simulink model "controller"  (R2021b)
settings: Solver=FixedStepAuto  StartTime=0.0  StopTime=inf  FixedStep=1/1000  RelTol=1e-3
libraries: simulink x2
settings Model: Creator=antonio  LastModifiedBy=antonio
settings OptimizationCC: DefaultUnderspecifiedDataType=single
settings ConfigComp: CovEnable=on  RecordCoverage=on  CovModelRefEnable=on

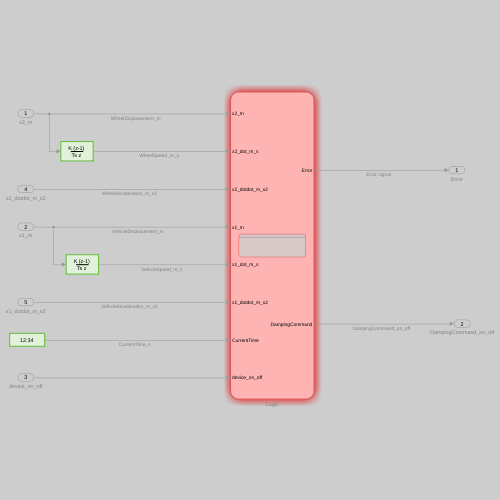
[thumbnail: Simulink's stored preview of the top-level diagram]
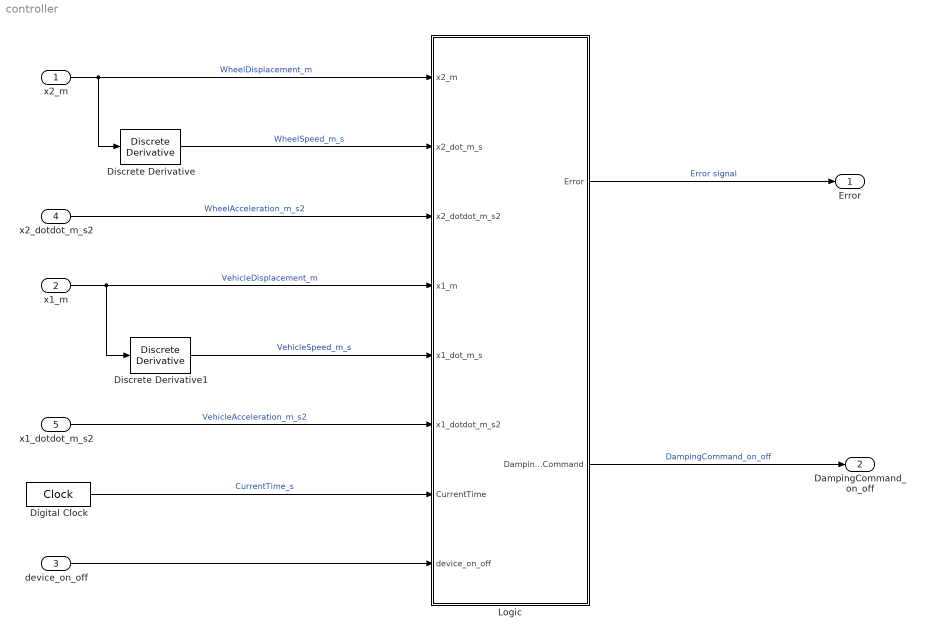
== system controller ==
  x2_m : Inport  OutDataTypeStr=double
  x1_m : Inport  Port=2
  device_on_off : Inport  Port=3
  x2_dotdot_m_s2 : Inport  Port=4  OutDataTypeStr=double
  x1_dotdot_m_s2 : Inport  Port=5  OutDataTypeStr=double
  Digital Clock : DigitalClock  SampleTime=1/100
  Discrete Derivative : simulink/Discrete/Discrete Derivative  gainval=1.0  ICPrevScaledInput=0.0  OutMin=[]  OutMax=[]  OutDataType=fixdt(1, 16)  OutScaling=2^-10  DoSatur=off
  Discrete Derivative1 : simulink/Discrete/Discrete Derivative  gainval=1.0  ICPrevScaledInput=0.0  OutMin=[]  OutMax=[]  OutDataType=fixdt(1, 16)  OutScaling=2^-10  DoSatur=off
  Logic : Stateflow chart  TreatAsAtomicUnit=on
  Error : Outport  OutDataTypeStr=double
  DampingCommand_on_off : Outport  Port=2  OutDataTypeStr=int8
  wires:
  x2_dotdot_m_s2/1 -> Logic/3(x2_dotdot_m_s2)  "WheelAcceleration_m_s2"
  Discrete Derivative/1 -> Logic/2(x2_dot_m_s)  "WheelSpeed_m_s"
  Digital Clock/1 -> Logic/7(CurrentTime)  "CurrentTime_s"
  x2_m/1 -> Logic/1(x2_m), Discrete Derivative/1  "WheelDisplacement_m"
  x1_dotdot_m_s2/1 -> Logic/6(x1_dotdot_m_s2)  "VehicleAcceleration_m_s2"
  Discrete Derivative1/1 -> Logic/5(x1_dot_m_s)  "VehicleSpeed_m_s"
  Logic/1(Error) -> Error/1  "Error signal"
  x1_m/1 -> Logic/4(x1_m), Discrete Derivative1/1  "VehicleDisplacement_m"
  Logic/2(DampingCommand) -> DampingCommand_on_off/1  "DampingCommand_on_off"
  device_on_off/1 -> Logic/8(device_on_off)

== stateflow chart controller/Logic ==
  state Device
    state DeviceOff
      entry:
      Error = 0;
      DampingCommand=0;
    state DeviceOn
      during:
      DecisionLogic();
      state Logic [parallel]
        settings: executionOrder=1
        state ControlLogic
          state HighDamping
            entry:
            DampingCommand=1;
          state LowDamping
            entry:
            DampingCommand=0;
          (default) -> HighDamping
          LowDamping -> HighDamping : [DampingStatus == "HiDamping"]
          HighDamping -> LowDamping : [DampingStatus == "LoDamping"]
        ControlLogic -> (junction 135)
        (junction 136) -> ControlLogic : {send(EStop,Warning)}
        (junction 135) -> (junction 136) : [CheckFaultSystem()]
      state Warning [parallel]
        settings: executionOrder=2
        state Running
        state Stop
          entry:
          Error=1;
          DampingCommand=1;
        (default) -> Running
        Running -> Stop : EStop
    (default) -> DeviceOff
    DeviceOn -> DeviceOff : [device_on_off==0]
    DeviceOff -> DeviceOn : [device_on_off==1]
  data: flag function_output; Error output double size=1 [0..1]; x2_m input double size=1; x2_dot_m_s input; x2_dotdot_m_s2 input double size=1; x1_m input double size=1; x1_dot_m_s input; DampingCommand output int8 size=1 [0..1]; x1_dotdot_m_s2 input double size=1; CurrentTime input double; DampingStatus local string; device_on_off input int8
  events: EStop local FUNCTION_CALL_EVENT
  function DecisionLogic:
    | function DecisionLogic
    | 
    | aVarTruthTableCondition_1 = false;
    | aVarTruthTableCondition_2 = false;
    | 
    | 
    | % High damping required
    | 
    | aVarTruthTableCondition_1 = logical((x1_dot_m_s-x2_dot_m_s)*x1_dot_m_s>=0 && Error<1);
    | 
    | % Low damping required
    | 
    | aVarTruthTableCondition_2 = logical((x1_dot_m_s-x2_dot_m_s)*x1_dot_m_s<0 && Error<1);
    | 
    | if (aVarTruthTableCondition_1)
    |     aFcnTruthTableAction_1();
    | elseif (aVarTruthTableCondition_2)
    |     aFcnTruthTableAction_2();
    | else % Default
    |     aFcnTruthTableAction_3();
    | end
    | 
    | function aFcnTruthTableAction_1()
    | 
    | % High damping coefficient
    | 
    | DampingStatus= "HiDamping";
    | 
    | function aFcnTruthTableAction_2()
    | 
    | % Low damping coefficient
    | 
    | DampingStatus = "LoDamping";
    | 
    | function aFcnTruthTableAction_3()
    | 
    | % Nothing
  function flag = CheckFaultSystem:
    | function flag = CheckFaultSystem
    | persistent tol old_x1_dotdot_m_s2 old_x1_m old_x2_m old_x2_dotdot_m_s2 timeChange Error_flag
    | 
    | if isempty(tol)
    |     tol = 1e-8;
    | end
    | 
    | if isempty(Error_flag)
    |     Error_flag = 0;
    | end
    | 
    | if isempty(old_x2_dotdot_m_s2)
    |     old_x2_dotdot_m_s2 = x2_dotdot_m_s2;
    | end
    | 
    | if isempty(old_x2_m)
    |     old_x2_m = x2_m;
    | end
    | 
    | if isempty(old_x1_dotdot_m_s2)
    |     old_x1_dotdot_m_s2 = x1_dotdot_m_s2;
    | end
    | 
    | if isempty(old_x1_m)
    |     old_x1_m = x1_m;
    | end
    | 
    | if isempty(timeChange)
    |     timeChange = CurrentTime;
    | end
    | 
    | if CurrentTime - timeChange >= 0.2 
    |     if abs(old_x1_m-x1_m)<=tol 
    |         Error_flag=1;
    |     elseif abs(old_x2_m-x2_m)<=tol 
    |         Error_flag=1;
    |     elseif abs(old_x1_dotdot_m_s2-x1_dotdot_m_s2)<=tol
    |         Error_flag=1;
    |     elseif abs(old_x2_dotdot_m_s2-x2_dotdot_m_s2)<=tol
    |         Error_flag=1;
    |     end
    |     timeChange = CurrentTime;
    |     old_x1_m = x1_m;
    |     old_x2_m = x2_m;
    |     old_x1_dotdot_m_s2 = x1_dotdot_m_s2;
    |     old_x2_dotdot_m_s2 = x2_dotdot_m_s2;
    |     %disp('%%%%%%%%%%%%%%%%%%%')
    | end
    | 
    | flag=Error_flag;
